simulink model "simlstabCtrl"  (R2016a)
settings: Solver=ode5  StartTime=0.0  StopTime=inf  FixedStep=0.001  RelTol=1e-3
undefined symbols (not defined in the file): Humusoft, MF644, robot
libraries: dcpctrl x5, sldrtlib x2, simulink x1
settings Model: SimulationMode=external  Creator=julianleland  LastModifiedBy=julianleland
settings HardwareCC: ProdBitPerLong=64  ProdLargestAtomicFloat=None  ProdHWDeviceType=Intel->x86-64  TargetBitPerLong=64  TargetBitPerPointer=64  TargetIntDivRoundTo=Zero  TargetEndianess=LittleEndian  TargetWordSize=64  TargetHWDeviceType=Intel->x86-64
settings RTWCC: SystemTargetFile=sldrt.tlc  TemplateMakefile=sldrt.tmf  Description=Simulink Desktop Real-Time  RTWCompilerOptimization=on
settings CodeAppCC: MaxIdLength=95
settings SimulinkDesktopRealTimeCC: TargetPreCompLibLocation=/Applications/MATLAB_R2016a.app/toolbox/sldrt/lib/maci64  TargetLangStandard=C89/C90 (ANSI)  SupportVariableSizeSignals=off

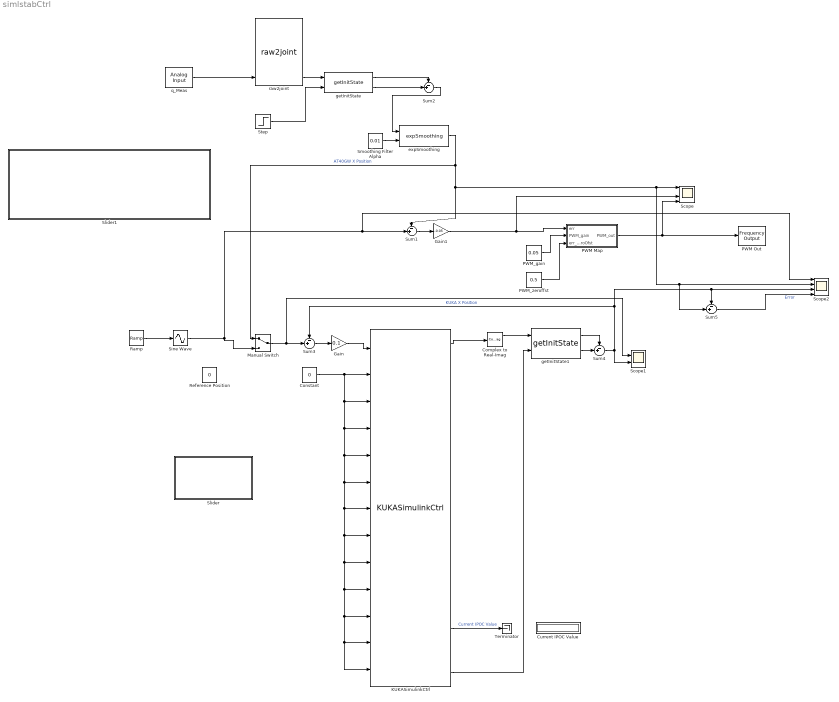
== system simlstabCtrl ==
  Complex to Real-Imag : ComplexToRealImag
  Constant : Constant  Value=0
  Current IPOC Value : Display
      settings: Floating=on
  Gain : Gain  Gain=0.1
  Gain1 : Gain  Gain=-0.05
  KUKASimulinkCtrl : dcpctrl/KUKASimulinkCtrl
      link override Triggered Subsystem/Stream Output: SampleTime=inf  MaxMissedTicks=10  ShowMissedTicks=on  YieldWhenWaiting=off  DrvName=Standard_Devices/UDP_Protocol  DrvAddress=27277  DrvOptions=[174338148 53453]  PortSizes=282  FormatString=repmat('%c',1,282)  ShowReady=on  ShowError=on  InitialValue=[]  FinalValue=[]
  Manual Switch : ManualSwitch
  PWM Map : Subsystem
  PWM Out : sldrtlib/Frequency Output  SampleTime=-1  MaxMissedTicks=10  ShowMissedTicks=off  YieldWhenWaiting=off  DrvName=Humusoft/MF644  DrvAddress=4294967295  DrvOptions=585  Channels=4  FrequencySource=1  Frequency=500  FrequencyFinalValue=[]  DutySource=2  Duty=0.5  DutyFinalValue=0.5
      settings: AttributesFormatString=Humusoft\nMF644 [auto]
  PWM_gain : Constant  Value=0.05
  PWM_zeroffst : Constant  Value=0.5
  Ramp : simulink/Sources/Ramp  slope=1  start=5  X0=0
  Reference Position : Constant  Value=0
  Scope : Scope  NumInputPorts=4
  Scope1 : Scope  NumInputPorts=2
  Scope2 : Scope  NumInputPorts=4
  Sine Wave : Sin  TimeSource=Use external signal  Amplitude=200  Frequency=0.3  SampleTime=0
  Slider : Subsystem  DialogController=hmiCreateDDGDialog  IsWebBlock=on  mask(MWDashboardBlock){webBlockId=ecd4f56a-e48d-4b8a-89b0-8b23b0e88b89, webBlockType=slider, ShowInLibBrowser=on, ShowInitialText=on, HMISrcModelName=ffpid_ctrl}
      mask prompts: webBlockId "WebBlock Id"; webBlockType "WebBlock Type"; HMISrcModelName "Source Model"
      mask Help: helpview([docroot '/mapfiles/simulink.map'], 'hmi_slider')
      mask Display:
      | if strcmp(get_param(bdroot(gcb),'BlockDiagramType'), 'library')
      |     image([(matlabroot) '/toolbox/simulink/hmi/icons/Slider.png']);
      | end
  Slider1 : Subsystem  DialogController=hmiCreateDDGDialog  IsWebBlock=on  mask(MWDashboardBlock){webBlockId=c64a29be-2d81-4e50-afc1-526ec20cd043, webBlockType=slider, ShowInLibBrowser=on, ShowInitialText=on, HMISrcModelName=ffpid_ctrl}
      mask prompts: webBlockId "WebBlock Id"; webBlockType "WebBlock Type"; HMISrcModelName "Source Model"
      mask Help: helpview([docroot '/mapfiles/simulink.map'], 'hmi_slider')
      mask Display:
      | if strcmp(get_param(bdroot(gcb),'BlockDiagramType'), 'library')
      |     image([(matlabroot) '/toolbox/simulink/hmi/icons/Slider.png']);
      | end
  Smoothing Filter Alpha : Constant  Value=0.01
  Step : Step  Time=0  SampleTime=0
  Sum{1..5} (5 alike) : Sum  Inputs=-+|
  Terminator : Terminator
  expSmoothing : dcpctrl/expSmoothing
  getInitState : dcpctrl/getInitState
  getInitState1 : dcpctrl/getInitState
  q_Meas : sldrtlib/Analog Input  SampleTime=-1  MaxMissedTicks=10  ShowMissedTicks=off  YieldWhenWaiting=off  DrvName=Humusoft/MF644  DrvAddress=4294967295  DrvOptions=585  Channels=5  RangeMode=1  VoltRange=1  DataType=1
      settings: AttributesFormatString=Humusoft\nMF644 [auto]
  raw2joint : dcpctrl/raw2joint
  wires:
  Step/1 -> getInitState/2
  q_Meas/1 -> raw2joint/4
  Sum3/1 -> Gain/1
  Gain/1 -> KUKASimulinkCtrl/1
  Constant/1 -> KUKASimulinkCtrl/3, KUKASimulinkCtrl/4, KUKASimulinkCtrl/5, KUKASimulinkCtrl/6, KUKASimulinkCtrl/7, KUKASimulinkCtrl/8, KUKASimulinkCtrl/9, KUKASimulinkCtrl/10, KUKASimulinkCtrl/11, KUKASimulinkCtrl/12, KUKASimulinkCtrl/13, KUKASimulinkCtrl/2
  KUKASimulinkCtrl/1 -> Complex to Real-Imag/1
  PWM_gain/1 -> PWM Map/2("PWM_gain ")
  Sum1/1 -> Gain1/1
  Sum2/1 -> expSmoothing/1
  Smoothing Filter Alpha/1 -> expSmoothing/2
  PWM Map/1(PWM_out) -> Scope/4, PWM Out/1
  getInitState/1 -> Sum2/1
  getInitState/2 -> Sum2/2
  raw2joint/4 -> getInitState/1
  Complex to Real-Imag/1 -> getInitState1/1
  getInitState1/2 -> Sum4/2
  getInitState1/1 -> Sum4/1
  Sum4/1 -> Sum5/1, Scope2/3, Sum3/1, Scope1/2  "KUKA X Position"
  KUKASimulinkCtrl/16 -> getInitState1/2
  Manual Switch/1 -> Scope1/1, Sum3/2
  expSmoothing/1 -> Manual Switch/1, Sum5/2, Scope2/2, Scope/1, Sum1/1  "AT40GW X Position"
  PWM_zeroffst/1 -> PWM Map/3(err_zeroOfst)
  Gain1/1 -> Scope/3, PWM Map/1(err)
  Sum5/1 -> Scope2/4  "Error"
  Sine Wave/1 -> Manual Switch/2, Scope2/1, Sum1/2
  Ramp/1 -> Sine Wave/1
  KUKASimulinkCtrl/14 -> Terminator/1  "Current IPOC Value"

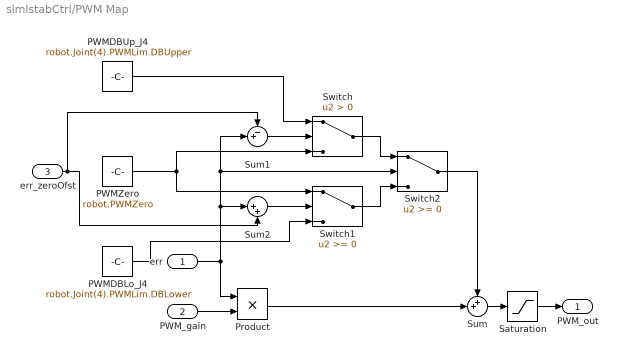
== system simlstabCtrl/PWM Map ==
  err : Inport
  "PWM_gain " : Inport  Port=2
  err_zeroOfst : Inport  Port=3
  PWMDBLo_J4 : Constant  Value=robot.Joint(4).PWMLim.DBLower
  PWMDBUp_J4 : Constant  Value=robot.Joint(4).PWMLim.DBUpper
  PWMZero : Constant  Value=robot.PWMZero
  Product : Product
  Saturation : Saturate  UpperLimit=robot.Joint(4).PWMLim.Max  LowerLimit=robot.Joint(4).PWMLim.Min
  Sum : Sum  Inputs=++|
  Sum1 : Sum  Inputs=-+|
  Sum2 : Sum  Inputs=|++
  Switch : Switch  Criteria=u2 > Threshold
  Switch1 : Switch
  Switch2 : Switch
  PWM_out : Outport
  wires:
  Sum/1 -> Saturation/1
  "PWM_gain "/1 -> Product/2
  err/1 -> Product/1, Sum2/1, Sum1/2, Switch2/2
  Product/1 -> Sum/2
  PWMDBUp_J4/1 -> Switch/1
  Saturation/1 -> PWM_out/1
  PWMDBLo_J4/1 -> Switch1/3
  PWMZero/1 -> Switch1/1, Switch/3
  Switch1/1 -> Switch2/3
  Switch/1 -> Switch2/1
  Switch2/1 -> Sum/1
  Sum1/1 -> Switch/2
  err_zeroOfst/1 -> Sum2/2, Sum1/1
  Sum2/1 -> Switch1/2

== system simlstabCtrl/Slider ==

== system simlstabCtrl/Slider1 ==
